simulink model "SERVER_COMMUNICATIONS_TEST"  (R2021b)
settings: Solver=FixedStepAuto  StartTime=0.0  StopTime=inf  FixedStep=0.03  RelTol=1e-3
undefined symbols (not defined in the file): CONTROL, f, MODEL
libraries: instrumentlib x16
settings Model: Creator=ae-dagbeyibor3  LastModifiedBy=ae-dagbeyibor3

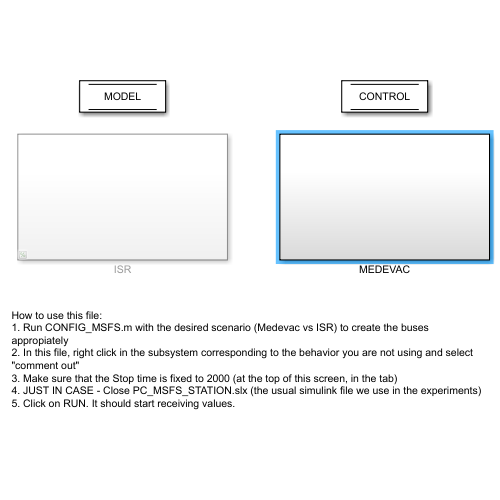
[thumbnail: Simulink's stored preview of the top-level diagram]
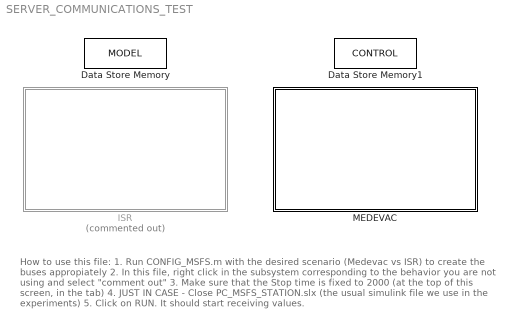
== system SERVER_COMMUNICATIONS_TEST ==
  note: How to use this file:
      | 1. Run CONFIG_MSFS.m with the desired scenario (Medevac vs ISR) to create the buses appropiately
      | 2. In this file, right click in the subsystem corresponding to the behavior you are not using and select "comment out"
      | 3. Make sure that the Stop time is fixed to 2000 (at the top of this screen, in the tab)
      | 4. JUST IN CASE - Close PC_MSFS_STATION.slx (the usual simulink file we use in the experiments)
      | 5. Click on RUN. It should start receiving values.
  Data Store Memory : DataStoreMemory  DataStoreName=MODEL  ReadBeforeWriteMsg=warning  WriteAfterWriteMsg=warning  WriteAfterReadMsg=warning  InitialValue=MODEL_INI  ShowAdditionalParam=off  OutDataTypeStr=Bus: MODEL_Bus
  Data Store Memory1 : DataStoreMemory  DataStoreName=CONTROL  ReadBeforeWriteMsg=warning  WriteAfterWriteMsg=warning  WriteAfterReadMsg=warning  InitialValue=CONTROL_INI  ShowAdditionalParam=off  OutDataTypeStr=Bus: CONTROL_Bus
  ISR : Subsystem  Commented=on
  MEDEVAC : Subsystem

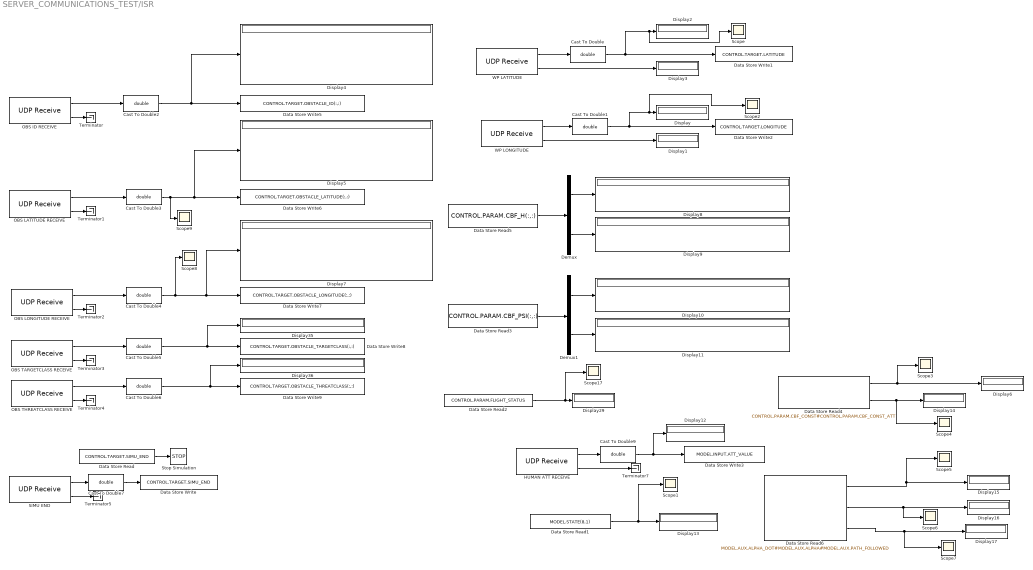
== system SERVER_COMMUNICATIONS_TEST/ISR ==
  Cast To Double{,1..7,9} (9 alike) : DataTypeConversion  OutDataTypeStr=double
  Data Store Read : DataStoreRead  DataStoreName=CONTROL  DataStoreElements=CONTROL.TARGET.SIMU_END  IndexOptions=Index vector (dialog)  Indices=1  OutputSizes=1
  Data Store Read1 : DataStoreRead  DataStoreName=MODEL  DataStoreElements=MODEL.STATE(8,1)  IndexOptions=Index vector (dialog)  Indices=1  OutputSizes=1
  Data Store Read2 : DataStoreRead  DataStoreName=CONTROL  DataStoreElements=CONTROL.PARAM.FLIGHT_STATUS  IndexOptions=Index vector (dialog)  Indices=1  OutputSizes=1
  Data Store Read3 : DataStoreRead  DataStoreName=CONTROL  DataStoreElements=CONTROL.PARAM.CBF_PSI(:,:)  IndexOptions=Index vector (dialog)  Indices=1  OutputSizes=1
  Data Store Read4 : DataStoreRead  DataStoreName=CONTROL  DataStoreElements=CONTROL.PARAM.CBF_CONST#CONTROL.PARAM.CBF_CONST_ATT  IndexOptions=Index vector (dialog)  Indices=1  OutputSizes=1
  Data Store Read5 : DataStoreRead  DataStoreName=CONTROL  DataStoreElements=CONTROL.PARAM.CBF_H(:,:)  IndexOptions=Index vector (dialog)  Indices=1  OutputSizes=1
  Data Store Read6 : DataStoreRead  DataStoreName=MODEL  DataStoreElements=MODEL.AUX.ALPHA_DOT#MODEL.AUX.ALPHA#MODEL.AUX.PATH_FOLLOWED  IndexOptions=Index vector (dialog)  Indices=1  OutputSizes=1
  Data Store Write : DataStoreWrite  DataStoreName=CONTROL  DataStoreElements=CONTROL.TARGET.SIMU_END  IndexOptions=Index vector (dialog)  Indices=1  OutputSizes=1
  Data Store Write1 : DataStoreWrite  DataStoreName=CONTROL  DataStoreElements=CONTROL.TARGET.LATITUDE  IndexOptions=Index vector (dialog)  Indices=1  OutputSizes=1
  Data Store Write2 : DataStoreWrite  DataStoreName=CONTROL  DataStoreElements=CONTROL.TARGET.LONGITUDE  IndexOptions=Index vector (dialog)  Indices=1  OutputSizes=1
  Data Store Write3 : DataStoreWrite  DataStoreName=MODEL  DataStoreElements=MODEL.INPUT.ATT_VALUE  IndexOptions=Index vector (dialog)  Indices=1  OutputSizes=1
  Data Store Write5 : DataStoreWrite  DataStoreName=CONTROL  DataStoreElements=CONTROL.TARGET.OBSTACLE_ID(:,:)  IndexOptions=Index vector (dialog)  Indices=1  OutputSizes=1
  Data Store Write6 : DataStoreWrite  DataStoreName=CONTROL  DataStoreElements=CONTROL.TARGET.OBSTACLE_LATITUDE(:,:)  IndexOptions=Index vector (dialog)  Indices=1  OutputSizes=1
  Data Store Write7 : DataStoreWrite  DataStoreName=CONTROL  DataStoreElements=CONTROL.TARGET.OBSTACLE_LONGITUDE(:,:)  IndexOptions=Index vector (dialog)  Indices=1  OutputSizes=1
  Data Store Write8 : DataStoreWrite  DataStoreName=CONTROL  DataStoreElements=CONTROL.TARGET.OBSTACLE_TARGETCLASS(:,:)  IndexOptions=Index vector (dialog)  Indices=1  OutputSizes=1
  Data Store Write9 : DataStoreWrite  DataStoreName=CONTROL  DataStoreElements=CONTROL.TARGET.OBSTACLE_THREATCLASS(:,:)  IndexOptions=Index vector (dialog)  Indices=1  OutputSizes=1
  Demux : Demux  Outputs=2
  Demux1 : Demux  Outputs=2
  Display{,1..17,29,35..36} (21 alike) : Display
  HUMAN ATT RECEIVE : instrumentlib/UDP Receive  Host=127.0.0.1  Port=7083  LocalPort=7082  EnablePortSharing=off  GetLatestData=off  DataSize="[1  1]"  DataType=double  ASCIIFormatting=%f,  Terminator=LF  ByteOrder=BigEndian  EnableBlockingMode=off  Timeout=10  SampleTime=-1  LocalAddress=127.0.0.1
  OBS ID RECEIVE : instrumentlib/UDP Receive  Host=127.0.0.1  Port=8081  LocalPort=8082  EnablePortSharing=off  GetLatestData=off  DataSize="[20   1]"  DataType=double  ASCIIFormatting=%f,  Terminator=LF  ByteOrder=BigEndian  EnableBlockingMode=off  Timeout=10  SampleTime=-1  LocalAddress=127.0.0.1
  OBS LATITUDE RECEIVE : instrumentlib/UDP Receive  Host=127.0.0.1  Port=8083  LocalPort=8084  EnablePortSharing=off  GetLatestData=off  DataSize="[20   1]"  DataType=double  ASCIIFormatting=%f,  Terminator=LF  ByteOrder=BigEndian  EnableBlockingMode=off  Timeout=10  SampleTime=-1  LocalAddress=127.0.0.1
  OBS LONGITUDE RECEIVE : instrumentlib/UDP Receive  Host=127.0.0.1  Port=8085  LocalPort=8086  EnablePortSharing=off  GetLatestData=off  DataSize="[20   1]"  DataType=double  ASCIIFormatting=%f,  Terminator=LF  ByteOrder=BigEndian  EnableBlockingMode=off  Timeout=10  SampleTime=-1  LocalAddress=127.0.0.1
  OBS TARGETCLASS RECEIVE : instrumentlib/UDP Receive  Host=127.0.0.1  Port=7087  LocalPort=7088  EnablePortSharing=off  GetLatestData=off  DataSize="[20   1]"  DataType=double  ASCIIFormatting=%f,  Terminator=LF  ByteOrder=BigEndian  EnableBlockingMode=off  Timeout=10  SampleTime=-1  LocalAddress=127.0.0.1
  OBS THREATCLASS RECEIVE : instrumentlib/UDP Receive  Host=127.0.0.1  Port=7089  LocalPort=7080  EnablePortSharing=off  GetLatestData=off  DataSize="[20   1]"  DataType=double  ASCIIFormatting=%f,  Terminator=LF  ByteOrder=BigEndian  EnableBlockingMode=off  Timeout=10  SampleTime=-1  LocalAddress=127.0.0.1
  SIMU END : instrumentlib/UDP Receive  Host=127.0.0.1  Port=7086  LocalPort=7084  EnablePortSharing=off  GetLatestData=off  DataSize=[1 1]  DataType=single  ASCIIFormatting=%f,  Terminator=LF  ByteOrder=BigEndian  EnableBlockingMode=off  Timeout=10  SampleTime=-1  LocalAddress=127.0.0.1
  Scope{,1..9,17} (11 alike) : Scope
  Stop Simulation : Stop
  Terminator{,1..5,7} (7 alike) : Terminator
  WP LATITUDE : instrumentlib/UDP Receive  Host=127.0.0.1  Port=8081  LocalPort=8080  EnablePortSharing=off  GetLatestData=off  DataSize=[1 1]  DataType=single  ASCIIFormatting=%f,  Terminator=LF  ByteOrder=BigEndian  EnableBlockingMode=off  Timeout=10  SampleTime=-1  LocalAddress=127.0.0.1
  WP LONGITUDE : instrumentlib/UDP Receive  Host=127.0.0.1  Port=8081  LocalPort=8088  EnablePortSharing=off  GetLatestData=off  DataSize=[1 1]  DataType=single  ASCIIFormatting=%f,  Terminator=LF  ByteOrder=BigEndian  EnableBlockingMode=off  Timeout=10  SampleTime=-1  LocalAddress=127.0.0.1
  wires:
  Cast To Double1/1 -> Scope2/1, Display/1, Data Store Write2/1
  Data Store Read2/1 -> Display29/1, Scope17/1
  Cast To Double2/1 -> Data Store Write5/1, Display4/1
  Cast To Double4/1 -> Scope8/1, Display7/1, Data Store Write7/1
  OBS THREATCLASS RECEIVE/1 -> Cast To Double6/1
  HUMAN ATT RECEIVE/1 -> Cast To Double9/1
  Data Store Read1/1 -> Display13/1, Scope1/1
  Data Store Read6/1 -> Scope5/1, Display15/1
  OBS LONGITUDE RECEIVE/1 -> Cast To Double4/1
  HUMAN ATT RECEIVE/2 -> Terminator7/1
  Data Store Read6/3 -> Display17/1, Scope7/1
  WP LONGITUDE/2 -> Display1/1
  WP LONGITUDE/1 -> Cast To Double1/1
  Cast To Double6/1 -> Display36/1, Data Store Write9/1
  OBS THREATCLASS RECEIVE/2 -> Terminator4/1
  Data Store Read4/2 -> Scope4/1, Display14/1
  WP LATITUDE/2 -> Display3/1
  OBS LATITUDE RECEIVE/2 -> Terminator1/1
  OBS ID RECEIVE/1 -> Cast To Double2/1
  Data Store Read6/2 -> Display16/1, Scope6/1
  Data Store Read3/1 -> Demux1/1
  SIMU END/1 -> Cast To Double7/1
  Cast To Double9/1 -> Display12/1, Data Store Write3/1
  Demux/1 -> Display8/1
  Cast To Double/1 -> Scope/1, Display2/1, Data Store Write1/1
  Data Store Read4/1 -> Display6/1, Scope3/1
  Cast To Double5/1 -> Display35/1, Data Store Write8/1
  OBS LONGITUDE RECEIVE/2 -> Terminator2/1
  WP LATITUDE/1 -> Cast To Double/1
  SIMU END/2 -> Terminator5/1
  OBS LATITUDE RECEIVE/1 -> Cast To Double3/1
  Cast To Double3/1 -> Scope9/1, Display5/1, Data Store Write6/1
  Cast To Double7/1 -> Data Store Write/1
  OBS TARGETCLASS RECEIVE/1 -> Cast To Double5/1
  Demux1/2 -> Display11/1
  Data Store Read/1 -> Stop Simulation/1
  Demux/2 -> Display9/1
  OBS TARGETCLASS RECEIVE/2 -> Terminator3/1
  Demux1/1 -> Display10/1
  Data Store Read5/1 -> Demux/1
  OBS ID RECEIVE/2 -> Terminator/1

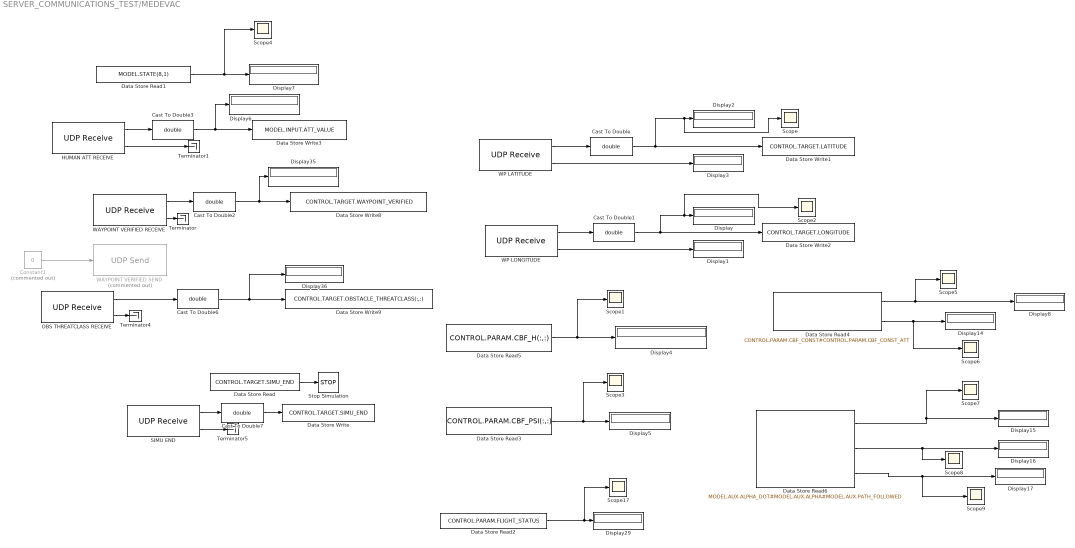
== system SERVER_COMMUNICATIONS_TEST/MEDEVAC ==
  Cast To Double{,1..3,6..7} (6 alike) : DataTypeConversion  OutDataTypeStr=double
  Constant1 : Constant  Commented=on  Value=0  SampleTime=-1
  Data Store Read : DataStoreRead  DataStoreName=CONTROL  DataStoreElements=CONTROL.TARGET.SIMU_END  IndexOptions=Index vector (dialog)  Indices=1  OutputSizes=1
  Data Store Read1 : DataStoreRead  DataStoreName=MODEL  DataStoreElements=MODEL.STATE(8,1)  IndexOptions=Index vector (dialog)  Indices=1  OutputSizes=1
  Data Store Read2 : DataStoreRead  DataStoreName=CONTROL  DataStoreElements=CONTROL.PARAM.FLIGHT_STATUS  IndexOptions=Index vector (dialog)  Indices=1  OutputSizes=1
  Data Store Read3 : DataStoreRead  DataStoreName=CONTROL  DataStoreElements=CONTROL.PARAM.CBF_PSI(:,:)  IndexOptions=Index vector (dialog)  Indices=1  OutputSizes=1
  Data Store Read4 : DataStoreRead  DataStoreName=CONTROL  DataStoreElements=CONTROL.PARAM.CBF_CONST#CONTROL.PARAM.CBF_CONST_ATT  IndexOptions=Index vector (dialog)  Indices=1  OutputSizes=1
  Data Store Read5 : DataStoreRead  DataStoreName=CONTROL  DataStoreElements=CONTROL.PARAM.CBF_H(:,:)  IndexOptions=Index vector (dialog)  Indices=1  OutputSizes=1
  Data Store Read6 : DataStoreRead  DataStoreName=MODEL  DataStoreElements=MODEL.AUX.ALPHA_DOT#MODEL.AUX.ALPHA#MODEL.AUX.PATH_FOLLOWED  IndexOptions=Index vector (dialog)  Indices=1  OutputSizes=1
  Data Store Write : DataStoreWrite  DataStoreName=CONTROL  DataStoreElements=CONTROL.TARGET.SIMU_END  IndexOptions=Index vector (dialog)  Indices=1  OutputSizes=1
  Data Store Write1 : DataStoreWrite  DataStoreName=CONTROL  DataStoreElements=CONTROL.TARGET.LATITUDE  IndexOptions=Index vector (dialog)  Indices=1  OutputSizes=1
  Data Store Write2 : DataStoreWrite  DataStoreName=CONTROL  DataStoreElements=CONTROL.TARGET.LONGITUDE  IndexOptions=Index vector (dialog)  Indices=1  OutputSizes=1
  Data Store Write3 : DataStoreWrite  DataStoreName=MODEL  DataStoreElements=MODEL.INPUT.ATT_VALUE  IndexOptions=Index vector (dialog)  Indices=1  OutputSizes=1
  Data Store Write8 : DataStoreWrite  DataStoreName=CONTROL  DataStoreElements=CONTROL.TARGET.WAYPOINT_VERIFIED  IndexOptions=Index vector (dialog)  Indices=1  OutputSizes=1
  Data Store Write9 : DataStoreWrite  DataStoreName=CONTROL  DataStoreElements=CONTROL.TARGET.OBSTACLE_THREATCLASS(:,:)  IndexOptions=Index vector (dialog)  Indices=1  OutputSizes=1
  Display{,1..8,14..17,29,35..36} (16 alike) : Display
  HUMAN ATT RECEIVE : instrumentlib/UDP Receive  Host=127.0.0.1  Port=7083  LocalPort=7082  EnablePortSharing=off  GetLatestData=off  DataSize="[1  1]"  DataType=double  ASCIIFormatting=%f,  Terminator=LF  ByteOrder=BigEndian  EnableBlockingMode=off  Timeout=10  SampleTime=-1  LocalAddress=127.0.0.1
  OBS THREATCLASS RECEIVE : instrumentlib/UDP Receive  Host=127.0.0.1  Port=7089  LocalPort=7080  EnablePortSharing=off  GetLatestData=off  DataSize="[1  1]"  DataType=double  ASCIIFormatting=%f,  Terminator=LF  ByteOrder=BigEndian  EnableBlockingMode=off  Timeout=10  SampleTime=-1  LocalAddress=127.0.0.1
  SIMU END : instrumentlib/UDP Receive  Host=127.0.0.1  Port=7086  LocalPort=7084  EnablePortSharing=off  GetLatestData=off  DataSize=[1 1]  DataType=single  ASCIIFormatting=%f,  Terminator=LF  ByteOrder=BigEndian  EnableBlockingMode=off  Timeout=10  SampleTime=-1  LocalAddress=127.0.0.1
  Scope{,1..9,17} (11 alike) : Scope
  Stop Simulation : Stop
  Terminator{,1,4..5} (4 alike) : Terminator
  WAYPOINT VERIFIED RECEIVE : instrumentlib/UDP Receive  Host=127.0.0.1  Port=7087  LocalPort=7088  EnablePortSharing=off  GetLatestData=off  DataSize="[1  1]"  DataType=double  ASCIIFormatting=%f,  Terminator=LF  ByteOrder=BigEndian  EnableBlockingMode=off  Timeout=10  SampleTime=-1  LocalAddress=127.0.0.1
  WAYPOINT VERIFIED SEND : instrumentlib/UDP Send  Commented=on  Host=127.0.0.1  Port=7088  LocalPort=7087  EnablePortSharing=off  ByteOrder=BigEndian  OutputDatagramPacketSize=512  EnableBlockingMode=on  LocalAddress=127.0.0.1
  WP LATITUDE : instrumentlib/UDP Receive  Host=127.0.0.1  Port=8081  LocalPort=8080  EnablePortSharing=off  GetLatestData=off  DataSize=[1 1]  DataType=single  ASCIIFormatting=%f,  Terminator=LF  ByteOrder=BigEndian  EnableBlockingMode=off  Timeout=10  SampleTime=-1  LocalAddress=127.0.0.1
  WP LONGITUDE : instrumentlib/UDP Receive  Host=127.0.0.1  Port=8081  LocalPort=8088  EnablePortSharing=off  GetLatestData=off  DataSize=[1 1]  DataType=single  ASCIIFormatting=%f,  Terminator=LF  ByteOrder=BigEndian  EnableBlockingMode=off  Timeout=10  SampleTime=-1  LocalAddress=127.0.0.1
  wires:
  Data Store Read6/2 -> Display16/1, Scope8/1
  Data Store Read6/3 -> Display17/1, Scope9/1
  SIMU END/2 -> Terminator5/1
  WP LONGITUDE/1 -> Cast To Double1/1
  Cast To Double7/1 -> Data Store Write/1
  Cast To Double/1 -> Data Store Write1/1, Display2/1, Scope/1
  Data Store Read4/2 -> Scope6/1, Display14/1
  Data Store Read1/1 -> Display7/1, Scope4/1
  Data Store Read/1 -> Stop Simulation/1
  WP LATITUDE/1 -> Cast To Double/1
  Data Store Read5/1 -> Display4/1, Scope1/1
  WAYPOINT VERIFIED RECEIVE/1 -> Cast To Double2/1
  Cast To Double6/1 -> Data Store Write9/1, Display36/1
  Cast To Double3/1 -> Display6/1, Data Store Write3/1
  Cast To Double1/1 -> Data Store Write2/1, Display/1, Scope2/1
  Data Store Read4/1 -> Display8/1, Scope5/1
  Data Store Read2/1 -> Scope17/1, Display29/1
  SIMU END/1 -> Cast To Double7/1
  WP LONGITUDE/2 -> Display1/1
  OBS THREATCLASS RECEIVE/1 -> Cast To Double6/1
  OBS THREATCLASS RECEIVE/2 -> Terminator4/1
  HUMAN ATT RECEIVE/2 -> Terminator1/1
  Data Store Read3/1 -> Display5/1, Scope3/1
  HUMAN ATT RECEIVE/1 -> Cast To Double3/1
  Constant1/1 -> WAYPOINT VERIFIED SEND/1
  Data Store Read6/1 -> Scope7/1, Display15/1
  Cast To Double2/1 -> Display35/1, Data Store Write8/1
  WAYPOINT VERIFIED RECEIVE/2 -> Terminator/1
  WP LATITUDE/2 -> Display3/1
